simulink model "my_chart"  (R2025b)
settings: Solver=FixedStepDiscrete  StartTime=0.0  StopTime=inf  FixedStep=0.02  RelTol=1e-3
libraries: simulink x2
settings Model: Creator=Huawei  LastModifiedBy=lolve
settings OptimizationCC: BlockReduction=off  UseDivisionForNetSlopeComputation=on  OptimizeBlockIOStorage=off

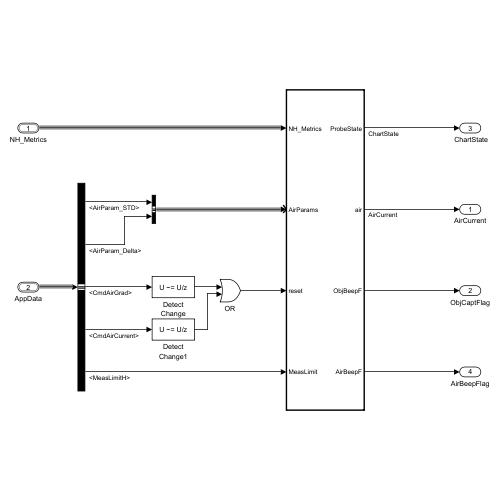
[thumbnail: Simulink's stored preview of the top-level diagram]
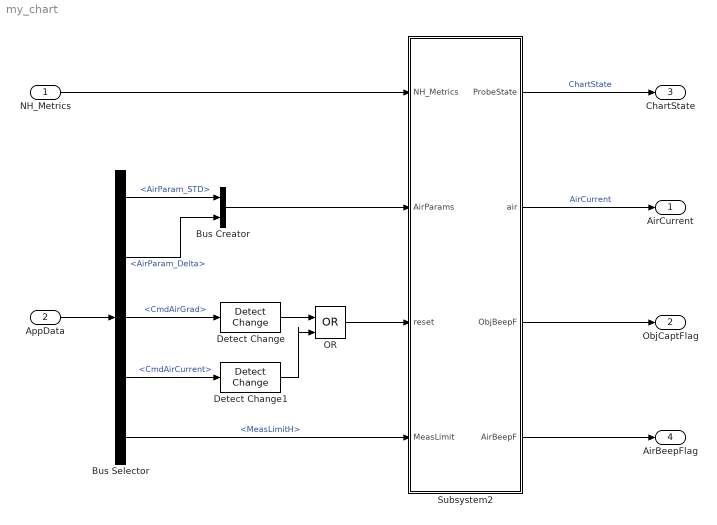
== system my_chart ==
  NH_Metrics : Inport  OutDataTypeStr=Bus: NH_MetricsBus_Type
  AppData : Inport  Port=2  OutDataTypeStr=Bus: FromAppBus_Type  PortDimensions=1
  Bus Creator : BusCreator  Inputs=2  OutDataTypeStr=Bus: AirParamsBus_Type
      settings: InheritFromInputs=off
  Bus Selector : BusSelector  OutputSignals=AirParam_STD,AirParam_Delta,CmdAirGrad,CmdAirCurrent,MeasLimitH
  Detect Change : simulink/Logic and Bit Operations/Detect Change  vinit=0  OutDataTypeStr=boolean
      settings: LibrarySourceBlock=|
      | hdlsllib/Logic and Bit
      | Operations/Detect
      | Change
  Detect Change1 : simulink/Logic and Bit Operations/Detect Change  vinit=0  OutDataTypeStr=boolean
      settings: LibrarySourceBlock=|
      | hdlsllib/Logic and Bit
      | Operations/Detect
      | Change
  OR : Logic  Operator=OR  IconShape=distinctive  AllPortsSameDT=off  OutDataTypeStr=boolean
  Subsystem2 : Subsystem  TreatAsAtomicUnit=on  SystemSampleTime=0.02
  AirCurrent : Outport
  ObjCaptFlag : Outport  Port=2
  " ChartState" : Outport  Port=3
  AirBeepFlag : Outport  Port=4
  wires:
  Bus Creator/1 -> Subsystem2/2(AirParams)
  Subsystem2/1(" ProbeState") -> " ChartState"/1  "ChartState"
  Subsystem2/3(ObjBeepF) -> ObjCaptFlag/1
  Subsystem2/2(air) -> AirCurrent/1  "AirCurrent"
  Detect Change/1 -> OR/1
  NH_Metrics/1 -> Subsystem2/1(NH_Metrics)
  AppData/1 -> Bus Selector/1
  Bus Selector/3 -> Detect Change/1  "<CmdAirGrad>"
  Bus Selector/4 -> Detect Change1/1  "<CmdAirCurrent>"
  Detect Change1/1 -> OR/2
  OR/1 -> Subsystem2/3(reset)
  Subsystem2/4(AirBeepF) -> AirBeepFlag/1
  Bus Selector/2 -> Bus Creator/2  "<AirParam_Delta>"
  Bus Selector/1 -> Bus Creator/1  "<AirParam_STD>"
  Bus Selector/5 -> Subsystem2/4(MeasLimit)  "<MeasLimitH>"

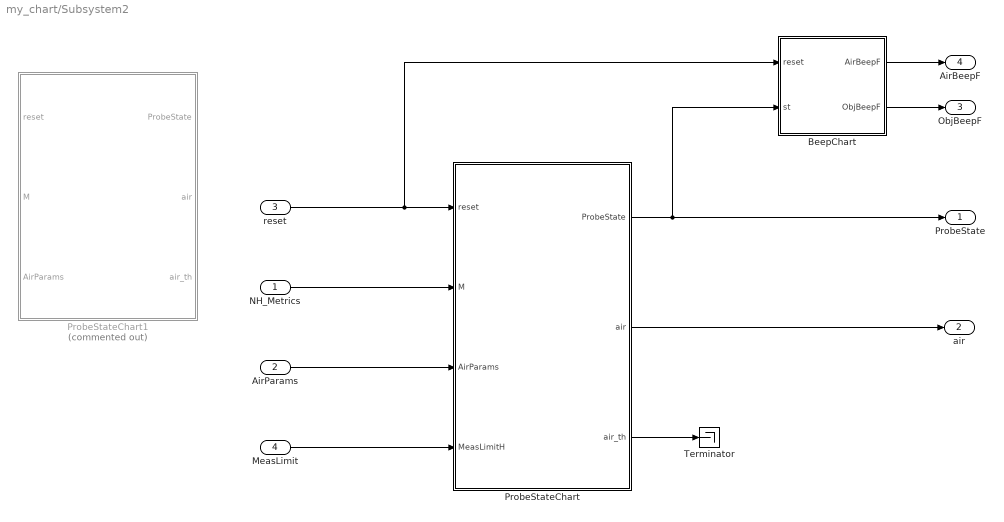
== system my_chart/Subsystem2 ==
  NH_Metrics : Inport  OutDataTypeStr=Bus: NH_MetricsBus_Type
  AirParams : Inport  Port=2  OutDataTypeStr=Bus: AirParamsBus_Type  PortDimensions=1
  reset : Inport  Port=3  OutDataTypeStr=boolean
  MeasLimit : Inport  Port=4  PortDimensions=1
  BeepChart : Stateflow chart  TreatAsAtomicUnit=on
      settings: PortSchema="{\"entries\":[{\"content\":{\"sides\":[{\"content\":{\"connectorIds\":[\"In2\",\"In1\"]},\"type\":\"ConnectorPlacement.EquallySpacedRectSide\",\"uuid\":\"9e8bd092-b09c-4138-9fd3-6d15d62c9049\"},{\"content\":{\"connectorIds\":[\"Out1\",\"Out2\"],\"side\":\"RIGHT\"},\"type\":\"ConnectorPlacement.EquallySpacedRectSide\",\"uuid\":\"35c69988-805e-4a20-aa0c-49e50e4389bb\"},{\"content\":{\"side\":\"TOP\"},\"type\":\"ConnectorPlacement.EquallySpacedRectSide\",\"uuid\":\"f72502a6-d622-4b29-9897-ab21c3e9277b\"}]},\"type\":\"ConnectorPlacement.EquallySpacedConnector\",\"uuid\":\"d6b9d547-7642-4069-b1d2-91f67ab057ec\"}],\"packageUris\":[\"http://schema.mathworks.com/mf0/Connector/R2020b\"],\"version\":\"1.0\"}"
  ProbeStateChart : Stateflow chart  Tag=myChart  TreatAsAtomicUnit=on  SystemSampleTime=0.02
      settings: PortSchema="{\"entries\":[{\"content\":{\"sides\":[{\"content\":{\"connectorIds\":[\"In2\",\"In3\",\"In1\",\"In4\"]},\"type\":\"ConnectorPlacement.EquallySpacedRectSide\",\"uuid\":\"3defb02b-9c2b-4794-b928-f4931306f746\"},{\"content\":{\"connectorIds\":[\"Out1\",\"Out2\",\"Out3\"],\"side\":\"RIGHT\"},\"type\":\"ConnectorPlacement.EquallySpacedRectSide\",\"uuid\":\"9e170d57-e22c-482a-ba3d-a140e52b56f4\"},{\"content\":{\"side\":\"TOP\"},\"type\":\"ConnectorPlacement.EquallySpacedRectSide\",\"uuid\":\"082772a8-38b1-4776-a8bf-0571bf977f0d\"}]},\"type\":\"ConnectorPlacement.EquallySpacedConnector\",\"uuid\":\"ce4fa0ae-f67e-4d06-bb19-0992ab93ff18\"}],\"packageUris\":[\"http://schema.mathworks.com/mf0/Connector/R2020b\"],\"version\":\"1.0\"}"
  ProbeStateChart1 : Stateflow chart  Tag=myChart  Commented=on  TreatAsAtomicUnit=on  SystemSampleTime=0.02
      settings: PortSchema="{\"entries\":[{\"content\":{\"sides\":[{\"content\":{\"connectorIds\":[\"In2\",\"In3\",\"In1\"]},\"type\":\"ConnectorPlacement.EquallySpacedRectSide\",\"uuid\":\"3defb02b-9c2b-4794-b928-f4931306f746\"},{\"content\":{\"connectorIds\":[\"Out1\",\"Out2\",\"Out3\"],\"side\":\"RIGHT\"},\"type\":\"ConnectorPlacement.EquallySpacedRectSide\",\"uuid\":\"9e170d57-e22c-482a-ba3d-a140e52b56f4\"},{\"content\":{\"side\":\"TOP\"},\"type\":\"ConnectorPlacement.EquallySpacedRectSide\",\"uuid\":\"082772a8-38b1-4776-a8bf-0571bf977f0d\"}]},\"type\":\"ConnectorPlacement.EquallySpacedConnector\",\"uuid\":\"ce4fa0ae-f67e-4d06-bb19-0992ab93ff18\"}],\"packageUris\":[\"http://schema.mathworks.com/mf0/Connector/R2020b\"],\"version\":\"1.0\"}"
  Terminator : Terminator
  " ProbeState" : Outport
  air : Outport  Port=2
  ObjBeepF : Outport  Port=3
  AirBeepF : Outport  Port=4
  wires:
  BeepChart/2(ObjBeepF) -> ObjBeepF/1
  reset/1 -> BeepChart/2(reset), ProbeStateChart/2(reset)
  AirParams/1 -> ProbeStateChart/1(AirParams)
  ProbeStateChart/1(" ProbeState") -> BeepChart/1(st), " ProbeState"/1
  ProbeStateChart/2(air) -> air/1
  NH_Metrics/1 -> ProbeStateChart/3(M)
  BeepChart/1(AirBeepF) -> AirBeepF/1
  ProbeStateChart/3(air_th) -> Terminator/1
  MeasLimit/1 -> ProbeStateChart/4(MeasLimitH)

== stateflow chart my_chart/Subsystem2/BeepChart ==
  state Continues
    entry:
    ObjBeepF = false;
    AirBeepF = false;
    WasOnObject = false;
    WasInMotion = false;
    note: Object
    note: Air
    (default) -> (junction 2)
    Continues -> (junction 2) [order 1]
    (junction 2) -> (junction 6) [order 1] : [st == pState.Moving]
    (junction 2) -> (junction 8) [order 2]
    (junction 6) -> (junction 18) : {WasInMotion = true;}
    (junction 18) -> (junction 8)
    (junction 8) -> (junction 20)
    (junction 20) -> (junction 22) [order 1] : [st == pState.ObjectUpdate]
    (junction 20) -> (junction 26) [order 2]
    (junction 22) -> (junction 24) : {WasOnObject = true;}
    (junction 24) -> (junction 28) [order 1] : [WasInMotion]
    (junction 24) -> (junction 32) [order 2]
    (junction 28) -> (junction 30) : {ObjBeepF = ~ObjBeepF;}
    (junction 32) -> (junction 30)
    (junction 30) -> (junction 35) : {WasInMotion = false;}
    (junction 35) -> (junction 26)
    (junction 26) -> (junction 39)
    (junction 39) -> (junction 41) [order 1] : [st == pState.AirUpdate]
    (junction 39) -> (junction 43) [order 2]
    (junction 41) -> (junction 45)
    (junction 45) -> (junction 47) [order 1] : [WasOnObject]
    (junction 47) -> (junction 51) : {AirBeepF = ~AirBeepF;}
    (junction 45) -> (junction 49) [order 2]
    (junction 49) -> (junction 51)
    (junction 51) -> (junction 54) : {WasOnObject = false; WasInMotion = true;}
    (junction 54) -> (junction 43)
  Continues -> Continues [order 1] : [reset]
  data: st input; reset input; WasInMotion local; WasOnObject local; AirBeepF output; ObjBeepF output

== stateflow chart my_chart/Subsystem2/ProbeStateChart1 ==
  state MainChart
    state pState [parallel]
      settings: executionOrder=2
      state NormOp
        state Air
          state AirUpdate
            entry, during:
            air_th = M.Nmean + AirParams.Delta;
            air = M.Nmean;
          state UnsteadyAir
          (default) -> UnsteadyAir
          UnsteadyAir -> AirUpdate : [update]
          AirUpdate -> UnsteadyAir : [~update]
        state ToAir
        state ToObject
        state Object
          state ObjectUpdate
          state UnsteadyObject
          (default) -> (junction 263)
          (junction 263) -> (junction 268) [order 1] : [update]
          (junction 263) -> UnsteadyObject [order 2]
          (junction 268) -> ObjectUpdate
          ObjectUpdate -> UnsteadyObject : [~update]
          UnsteadyObject -> ObjectUpdate : [update]
        (default) -> Air
        Air -> ToObject : [action == down || ~InAir]
        ToAir -> Air [order 2] : [action == stop && InAir]
        ToAir -> ToObject [order 1] : [action == down]
        ToObject -> ToAir [order 1] : [action == up]
        Object -> ToAir [order 1] : [action == up ||...
            | InAir]
        ToAir -> Object [order 3] : [action == stop && ~InAir]
        ToObject -> Object [order 2] : [action == stop]
        Object -> ToObject [order 2] : [action == down]
      state AirTimeout
      (default) -> NormOp
      NormOp -> AirTimeout : [IsAirTimeout == true]
    state pAirWatchDog [parallel]
      settings: executionOrder=3
      state WD_Active
      state AirTimeoutTrig
        entry:
        IsAirTimeout = true;
      (default) -> WD_Active
      WD_Active -> AirTimeoutTrig [order 1] : after(10, sec)
      WD_Active -> WD_Active [order 2] : [in(pState.NormOp.Air.AirUpdate)]
    state pActionEntry [parallel]
      settings: executionOrder=1
      state pcond
        entry:
        Hstd_th = 0;
        air = M.Nlast;
        air_th = M.Nlast + AirParams.Delta;
        InAir = true;
        update = false;
        IsAirTimeout = false;
        %------------------------------------
        during:
        Hstd_th = abs( M.Hlast) * 0.005 +0.5;
        (default) -> (junction 297)
        pcond -> (junction 297)
        (junction 297) -> (junction 173) : {action = stop;}
        (junction 173) -> (junction 175) [order 1] : [M.Nmean < air_th]
        (junction 173) -> (junction 146) [order 2] : {InAir = false;}
        (junction 175) -> (junction 177) : {InAir = true;}
        (junction 146) -> (junction 151) [order 1] : [M.Hstd <= Hstd_th]
        (junction 177) -> (junction 151) [order 1] : [M.Nstd <= AirParams.STD]
        (junction 146) -> (junction 319) [order 2] : {update = false;}
        (junction 151) -> (junction 155) : {update = true;}
        (junction 177) -> (junction 300) [order 2] : {update = false;}
        (junction 319) -> (junction 323) [order 1] : [M.Hlast > 3121]
        (junction 319) -> (junction 272) [order 2]
        (junction 323) -> (junction 325) : {action = unknown;}
        (junction 272) -> (junction 3) [order 1] : [M.Hdif < -Hstd_th  *2]
        (junction 3) -> (junction 6) : {action = down;}
        (junction 272) -> (junction 273) [order 2]
        (junction 6) -> (junction 273)
        (junction 273) -> (junction 275)
        (junction 275) -> (junction 8) [order 1] : [M.Hdif >  Hstd_th *2]
        (junction 8) -> (junction 10) : {action = up;}
        (junction 275) -> (junction 277) [order 2]
        (junction 10) -> (junction 277)
        (junction 277) -> (junction 321)
        (junction 325) -> (junction 321)
        (junction 321) -> (junction 199)
        (junction 300) -> (junction 155)
        (junction 155) -> (junction 199)
      (default) -> pcond
  (default) -> MainChart
  MainChart -> MainChart : [reset]
  data: AirParams input; down constant double =1; up constant double =-1; stop constant double =0; action local; ProbeState output Enum: pState; air output; InAir local; update local; reset input; M input; IsAirTimeout local; Hstd_th local; air_th output; unknown constant double =2

== stateflow chart my_chart/Subsystem2/ProbeStateChart ==
  state MainChart
    state pState [parallel]
      settings: executionOrder=2
      state NormOp
        state Air
          state AirUpdate
            entry, during:
            air_th = M.Nmean + AirParams.Delta;
            air = M.Nmean;
          state UnsteadyAir
          (default) -> UnsteadyAir
          UnsteadyAir -> AirUpdate : [update]
          AirUpdate -> UnsteadyAir : [~update]
        state Moving
        state Object
          state ObjectUpdate
          state UnsteadyObject
          (default) -> (junction 263)
          (junction 263) -> (junction 268) [order 1] : [update]
          (junction 263) -> UnsteadyObject [order 2]
          (junction 268) -> ObjectUpdate
          ObjectUpdate -> UnsteadyObject : [~update]
          UnsteadyObject -> ObjectUpdate : [update]
        (default) -> Air
        Air -> Moving : [action == moving || ~InAir]
        Moving -> Air [order 1] : [action == stop && InAir]
        Moving -> Object [order 2] : [action == stop && ~InAir]
        Object -> Moving : [action == moving || InAir]
      state AirTimeout
      (default) -> NormOp
      NormOp -> AirTimeout : [IsAirTimeout == true]
    state pAirWatchDog [parallel]
      settings: executionOrder=3
      state WD_Active
      state AirTimeoutTrig
        entry:
        IsAirTimeout = true;
      (default) -> WD_Active
      WD_Active -> AirTimeoutTrig [order 1] : after(10, sec)
      WD_Active -> WD_Active [order 2] : [in(pState.NormOp.Air.AirUpdate)]
    state pActionEntry [parallel]
      settings: executionOrder=1
      state pcond
        entry:
        Hstd_th = 0;
        air = M.Nlast;
        air_th = M.Nlast + AirParams.Delta;
        InAir = true;
        update = false;
        IsAirTimeout = false;
        %------------------------------------
        during:
        Hstd_th = abs( M.Hlast) * 0.005 +0.5;
        (default) -> (junction 297)
        pcond -> (junction 297)
        (junction 297) -> (junction 173) : {action = stop;}
        (junction 173) -> (junction 175) [order 1] : [M.Nmean < air_th]
        (junction 173) -> (junction 146) [order 2] : {InAir = false;}
        (junction 175) -> (junction 177) : {InAir = true;}
        (junction 146) -> (junction 151) [order 1] : [M.Hstd <= Hstd_th]
        (junction 177) -> (junction 151) [order 1] : [M.Nstd <= AirParams.STD]
        (junction 146) -> (junction 319) [order 2] : {update = false;}
        (junction 151) -> (junction 155) : {update = true;}
        (junction 177) -> (junction 300) [order 2] : {update = false;}
        (junction 319) -> (junction 323) [order 1] : [M.Hlast > MeasLimitH]
        (junction 319) -> (junction 275) [order 2]
        (junction 323) -> (junction 8)
        (junction 275) -> (junction 8) [order 1] : [abs( M.Hdif) >  Hstd_th *2]
        (junction 8) -> (junction 10) : {action = moving;}
        (junction 275) -> (junction 277) [order 2]
        (junction 10) -> (junction 277)
        (junction 277) -> (junction 199)
        (junction 300) -> (junction 155)
        (junction 155) -> (junction 199)
      (default) -> pcond
  (default) -> MainChart
  MainChart -> MainChart : [reset]
  data: AirParams input; stop constant double =0; action local; ProbeState output Enum: pState; air output; InAir local; update local; reset input; M input; IsAirTimeout local; Hstd_th local; air_th output; moving constant double =2; MeasLimitH input
